simulink model "without_absorber"  (R2022b)
settings: Solver=VariableStepAuto  StartTime=0.0  StopTime=10.0  RelTol=1e-3
values from neighbouring files (symbols this model uses):
  F_amp = m*e*w^2    (= 41.1233516712)    [A_plus.m]
  k1 = 38000    [A_plus.m]
  m1 = 0.55    [A_plus.m]
  w = 2500*2*pi/60    (= 261.799387799)    [A_plus.m]
settings Model: Creator=a7mad  LastModifiedBy=a7mad

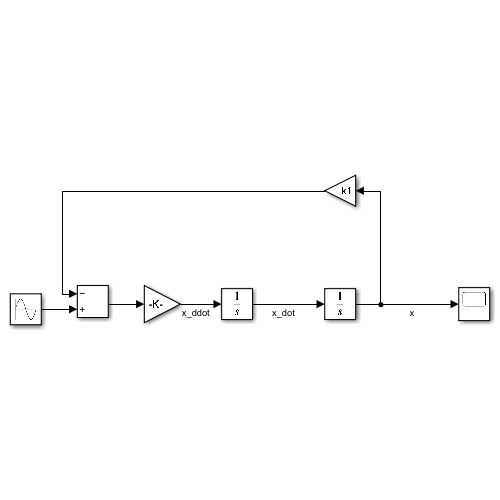
[thumbnail: Simulink's stored preview of the top-level diagram]
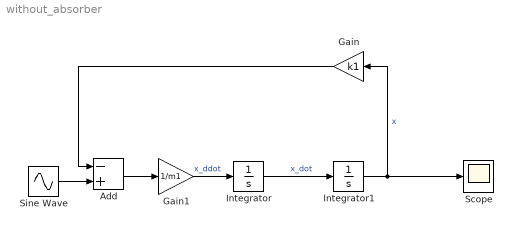
== system without_absorber ==
  Add : Sum  Inputs=-+
  Gain : Gain  Gain=k1
  Gain1 : Gain  Gain=1/m1
  Integrator : Integrator
  Integrator1 : Integrator
  Scope : Scope
  Sine Wave : Sin  Amplitude=F_amp  Frequency=w  SampleTime=0
  wires:
  Integrator/1 -> Integrator1/1  "x_dot"
  Integrator1/1 -> Scope/1, Gain/1  "x"
  Gain1/1 -> Integrator/1  "x_ddot"
  Add/1 -> Gain1/1
  Gain/1 -> Add/1
  Sine Wave/1 -> Add/2
